simulink library "JavaBoxLibrary"  (Simulink 6.0)
settings: Solver=ode45  StartTime=0.0  StopTime=10.0  RelTol=1e-3
settings Model: LastModifiedBy=BrownM5

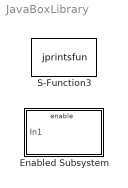
== system JavaBoxLibrary ==
  Enabled Subsystem : Subsystem  TreatAsAtomicUnit=on  mask(Java Display Box){dev=1, fmt1=, fmt2=, fmt3=, fmt4=, fmt5=, fmt6=, fmt7=}
      mask prompts: dev "Display number"; fmt1 "Initialization format"; fmt2 "Update leader format"; fmt3 "Update numeric format"; fmt4 "Update trailer format"; fmt5 "Termination leader format"; fmt6 "Termination numeric format"; fmt7 "Termination trailer format"
      mask help:
      | Displays formatted text and numeric data to an editable Java window.
      | "Display Number" is a positive integer which specifies the Java window to receive the formatted output. Seven format strings control the appearance of the output during block initialization, update, and termination.  These strings can contain any combination of text and format specifiers acceptable to the Matlab FPRINTF function.
      |
      | See HELP for more information.
      mask Help:
      | <HTML>
      | 
      | <head>
      | <TITLE>Java Display Box</TITLE>
      | </head>
      | 
      | <body>
      | 
      | <h2>Function</h2>
      | Displays formatted text and numeric data to an editable Java window.
      | "Display Number" is a positive integer which specifies the Java window to receive the
      | formatted output. Seven format strings control the appearance of the output during
      | block initialization, update, and termination.  These strings can contain any combination
      | of text and format specifiers acceptable to the Matlab FPRINTF function.
      | 
      | <h2>Inputs</h2>
      | Java Display Box accepts any Simulink scalar, vector, or matrix signal.  The signal
      | must be real and double precision.  It is up to the user to perform data type conversion
      | (e.g. int8 to double) and to break apart complex signals into separate real and
      | imaginary parts.  This function will accept multiplexed signals and bus signals.  When
      | displaying matrix signals, Java Display Box will access the matrix data in columnwise
      | order, so you may need to transpose the matrix to display the matrix in it's natural
      | orientation.
      | 
      | <h2>Parameters</h2>
      | 
      | <h3>Display Number:</h3>
      | The display number is a numeric identifier for each active Java Display Box.  Any
      | positive integer greater than zero is acceptable.  If you want the outputs to go do
      | different windows, use differerent Display Numbers for each Java Display Box.
      | You can send multiple signals to the same window by using the same Display
      | Number.  In this case, the order in which the output is written to the box depends on
      | Simulink's execution order, called Sorted Order.  You can force multiple outputs to be
      | displayed in any desired sequence by overriding Simulink's Sorted Order using the
      | block priority property.  To change a Java Display Box priority, right-click the Java Box,
      | select Block  Properties, and enter a numeric value for Block Priority.  The lower the
      | number, the higher the priority, so a good rule of thumb is to assign priorities in the
      | order in which  you want the output to appear in the Java Display Box.
      | <br><br>
      | Note that multiple models share the same set of Java Display Boxes, so if you have
      | more than one model open and those models all access Display Box 1, then the
      | outputs from both models will appear in the same display window.
      | <br><br>
      | If you set the Display Number to -1, the outputs will go to the "standard output", normally
      | the Matlab command window.  A Display Number of -2 will send output to "standard
      | error", and a Display Number consisting of a valid handle to an open file will cause
      | the output to be written to the file.  The user is responsible for opening and closing
      | the file, and passing the file handle to Java Display Box.
      | 
      | <h3>Initialization Format:</h3>
      | The initialization format string is written once during model initialization.  Enter any valid
      | format string (without quotation marks!).  Note that during initialization, the input signal
      | values are generally undefined, so it is not possible to display numeric values of input
      | signals during initialization.  The Initialization Format is generally useful for printing
      | column headers or other delimiters to mark the beginning of a simulation run.  If you
      | don't want any initialization format, leave this field completely blank (i.e. no spaces or
      | other characters).
      | 
      | <h3>Update Format:</h3>
      | The update format strings consist of three parts:  Leader Format, Numeric Format, and
      | Trailer Format.  At each Simulink update time step, the Leader Format is first written
      | once.  Then the Numeric Format is applied to the input signal data, and repeated as
      | necessary to display all of the inputs.  Finally, the Trailer Format is written.  Typically,
      | the Leader Format contains textual information, such as 'Signal Amplitude = ', the
      | Numeric Format contains number formatting strings such as '%6.4f', and the Trailer
      | Format contains units and carriage controls such as '(volts)\n'.
      | 
      | <br><br>Be carefull!  If you have a lengthy simulation, or one that involves many time
      | steps, you can overrun the display memory.  If this is a possibility, consider using a
      | downsampler block in front of the Java Display Box, or enclose it in a triggered
      | subsystem so that only selected time samples are displayed.  If you don't want a
      | Leader, Numeric, or Trailer format, leave the field completely blank.
      | 
      | <h3>Termination Format:</h3>
      | The termination format string consists of three parts:  Leader Format, Numeric Format,
      | and Trailer Format.   These three formats are applied once at the end of a Simulink
      | simulation run.   First, the Leader Format is written once.  Then the Numeric Format is
      | applied to the input signal data, and repeated as necessary to display all of the inputs.
      | Finally, the Trailer Format is written.  Typically, the Leader Format contains textual
      | information, such as 'Signal Amplitude = ', the Numeric Format contains number
      | formatting strings such as '%6.4f', and the Trailer Format contains units and carriage
      | controls such as '(volts)\n'.  These formats are useful if you only want to display the
      | final values of signals at the end of simulation.  You can also use these fields to print
      | summary information, or model termination status.  If you don't want a Leader,
      | Numeric, or Trailer format, leave the field completely blank.
      | 
      | <h2>Java Display Box Menu:</h2>
      | These are fairly self-explanatory.  See HELP on the Java Box pulldown menu for more information.
      | 
      | </body>
      | 
      | </html>
      mask Display: fprintf('Enabled\nJava Box %d',dev)
  S-Function3 : S-Function  Priority=4  FunctionName=jprintsfun  Parameters=dev,{fmt1,fmt2,fmt3,fmt4,fmt5,fmt6,fmt7}  mask(Java Display Box){dev=1, fmt1=, fmt2=, fmt3=, fmt4=, fmt5=, fmt6=, fmt7=}
      mask prompts: dev "Display number"; fmt1 "Initialization format"; fmt2 "Update leader format"; fmt3 "Update numeric format"; fmt4 "Update trailer format"; fmt5 "Termination leader format"; fmt6 "Termination numeric format"; fmt7 "Termination trailer format"
      mask help:
      | Displays formatted text and numeric data to an editable Java window.
      | "Display Number" is a positive integer which specifies the Java window to receive the formatted output. Seven format strings control the appearance of the output during block initialization, update, and termination.  These strings can contain any combination of text and format specifiers acceptable to the Matlab FPRINTF function.
      |
      | See HELP for more information.
      mask Help:
      | <HTML>
      | 
      | <head>
      | <TITLE>Java Display Box</TITLE>
      | </head>
      | 
      | <body>
      | 
      | <h2>Function</h2>
      | Displays formatted text and numeric data to an editable Java window.
      | "Display Number" is a positive integer which specifies the Java window to receive the
      | formatted output. Seven format strings control the appearance of the output during
      | block initialization, update, and termination.  These strings can contain any combination
      | of text and format specifiers acceptable to the Matlab FPRINTF function.
      | 
      | <h2>Inputs</h2>
      | Java Display Box accepts any Simulink scalar, vector, or matrix signal.  The signal
      | must be real and double precision.  It is up to the user to perform data type conversion
      | (e.g. int8 to double) and to break apart complex signals into separate real and
      | imaginary parts.  This function will accept multiplexed signals and bus signals.  When
      | displaying matrix signals, Java Display Box will access the matrix data in columnwise
      | order, so you may need to transpose the matrix to display the matrix in it's natural
      | orientation.
      | 
      | <h2>Parameters</h2>
      | 
      | <h3>Display Number:</h3>
      | The display number is a numeric identifier for each active Java Display Box.  Any
      | positive integer greater than zero is acceptable.  If you want the outputs to go do
      | different windows, use differerent Display Numbers for each Java Display Box.
      | You can send multiple signals to the same window by using the same Display
      | Number.  In this case, the order in which the output is written to the box depends on
      | Simulink's execution order, called Sorted Order.  You can force multiple outputs to be
      | displayed in any desired sequence by overriding Simulink's Sorted Order using the
      | block priority property.  To change a Java Display Box priority, right-click the Java Box,
      | select Block  Properties, and enter a numeric value for Block Priority.  The lower the
      | number, the higher the priority, so a good rule of thumb is to assign priorities in the
      | order in which  you want the output to appear in the Java Display Box.
      | <br><br>
      | Note that multiple models share the same set of Java Display Boxes, so if you have
      | more than one model open and those models all access Display Box 1, then the
      | outputs from both models will appear in the same display window.
      | <br><br>
      | If you set the Display Number to -1, the outputs will go to the "standard output", normally
      | the Matlab command window.  A Display Number of -2 will send output to "standard
      | error", and a Display Number consisting of a valid handle to an open file will cause
      | the output to be written to the file.  The user is responsible for opening and closing
      | the file, and passing the file handle to Java Display Box.
      | 
      | <h3>Initialization Format:</h3>
      | The initialization format string is written once during model initialization.  Enter any valid
      | format string (without quotation marks!).  Note that during initialization, the input signal
      | values are generally undefined, so it is not possible to display numeric values of input
      | signals during initialization.  The Initialization Format is generally useful for printing
      | column headers or other delimiters to mark the beginning of a simulation run.  If you
      | don't want any initialization format, leave this field completely blank (i.e. no spaces or
      | other characters).
      | 
      | <h3>Update Format:</h3>
      | The update format strings consist of three parts:  Leader Format, Numeric Format, and
      | Trailer Format.  At each Simulink update time step, the Leader Format is first written
      | once.  Then the Numeric Format is applied to the input signal data, and repeated as
      | necessary to display all of the inputs.  Finally, the Trailer Format is written.  Typically,
      | the Leader Format contains textual information, such as 'Signal Amplitude = ', the
      | Numeric Format contains number formatting strings such as '%6.4f', and the Trailer
      | Format contains units and carriage controls such as '(volts)\n'.
      | 
      | <br><br>Be carefull!  If you have a lengthy simulation, or one that involves many time
      | steps, you can overrun the display memory.  If this is a possibility, consider using a
      | downsampler block in front of the Java Display Box, or enclose it in a triggered
      | subsystem so that only selected time samples are displayed.  If you don't want a
      | Leader, Numeric, or Trailer format, leave the field completely blank.
      | 
      | <h3>Termination Format:</h3>
      | The termination format string consists of three parts:  Leader Format, Numeric Format,
      | and Trailer Format.   These three formats are applied once at the end of a Simulink
      | simulation run.   First, the Leader Format is written once.  Then the Numeric Format is
      | applied to the input signal data, and repeated as necessary to display all of the inputs.
      | Finally, the Trailer Format is written.  Typically, the Leader Format contains textual
      | information, such as 'Signal Amplitude = ', the Numeric Format contains number
      | formatting strings such as '%6.4f', and the Trailer Format contains units and carriage
      | controls such as '(volts)\n'.  These formats are useful if you only want to display the
      | final values of signals at the end of simulation.  You can also use these fields to print
      | summary information, or model termination status.  If you don't want a Leader,
      | Numeric, or Trailer format, leave the field completely blank.
      | 
      | <h2>Java Display Box Menu:</h2>
      | These are fairly self-explanatory.  See HELP on the Java Box pulldown menu for more information.
      | 
      | </body>
      | 
      | </html>
      mask Display: disp(['Java Box ',num2str(dev)])

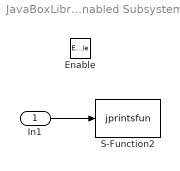
== system JavaBoxLibrary/Enabled Subsystem ==
  In1 : Inport  Port=1  LatchInput=off
  Enable : EnablePort
  S-Function2 : S-Function  Priority=4  FunctionName=jprintsfun  Parameters=dev,{fmt1,fmt2,fmt3,fmt4,fmt5,fmt6,fmt7}
  wires:
  In1/1 -> S-Function2/1
